simulink model "model"  (Simulink 7.7)
settings: Solver=ode45  StartTime=0.0  StopTime=2500000  FixedStep=0.01  RelTol=1e-3
undefined symbols (not defined in the file): des_figposition
libraries: simeventssink1 x5, simeventsgenerators1 x3, simeventsattributes2 x2, simeventsqueue1 x1, simeventsserver1 x1, simeventsrouting1 x1
settings Model: Creator=Yulia  ModifiedByFormat=Yuli  LastModifiedBy=Yuli  ModifiedComment=Yulia -- Yulia -- Version 1.8
settings Model: ModifiedHistory=|
  | Yulia -- Yulia -- Version 1.8
  | 
  | 
  | Yulia -- Yulia -- Version 1.7
settings OptimizationCC: SimCompilerOptimization=On
settings SimEventsCC: propDiagAttribOutput=1  propDiagFcnCallOutput=1  propDiagStatOutput=0

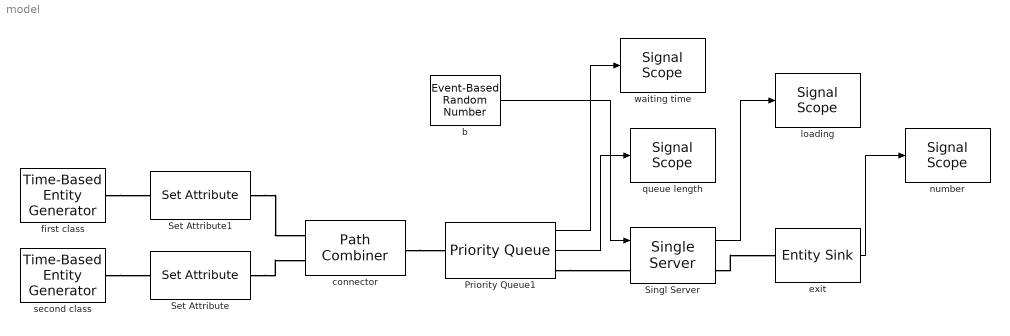
== system model ==
  Priority Queue1 : simeventsqueue1/Priority Queue  Priority=1  SystemSampleTime=-1  Capacity=inf  SortingAttributeName=ServiceTime  SortingDirection=Descending  EnableTOPort=off  StatNumberDeparted=Off  StatNumberInBlock=Off  StatPendingEntity=Off  StatAverageWait=On  StatAverageQueueLength=On  StatNumberTimedout=Off
      settings: AttributesFormatString=Sorting direction =\n%<SortingDirection>
  Set Attribute : simeventsattributes2/Set Attribute  Priority=1  SystemSampleTime=-1  AttributeFrom=Dialog  AttributeName=ServiceTime  AttributeTreatAsVector=1  AttributeValue=2  AttributeCreate=on  StatNumberDeparted=Off  EvaluatedAttributeValue={2}
      settings: AttributesFormatString=ServiceTime = 2\nSwitch = 2
  Set Attribute1 : simeventsattributes2/Set Attribute  Priority=1  SystemSampleTime=-1  AttributeFrom=Dialog  AttributeName=ServiceTime  AttributeTreatAsVector=1  AttributeValue=1  AttributeCreate=on  StatNumberDeparted=Off  EvaluatedAttributeValue={1}
      settings: AttributesFormatString=ServiceTime = 1\nSwitch = 1
  Singl Server : simeventsserver1/Single Server  SystemSampleTime=-1  ServiceTimeFrom=Signal port t  ServiceTime=1  AttributeName=ServiceTime  PriorityServiceCompletion=500  PermitPreemption=off  SortingAttributeName=PriorityAttributeName  SortingDirection=Ascending  WriteToAttribute=off  ResidualAttributeName=ResidualServiceTime  CreateAttribute=on  EnableTOPort=off  StatNumberDeparted=Off  StatNumberInBlock=Off  StatNumberPreempted=Off  StatPendingEntity=Off  StatAverageWait=Off  StatUtilization=On  StatNumberTimedout=Off
  b : simeventsgenerators1/Signal Generators/Event-Based Random Number  SystemSampleTime=-1  distribution=Exponential  meanExp=1  minUnif=1  maxUnif=1  pOneBern=0.25  pSuccessBino=0.5  numTrialBino=1  meanNorm=0  stdNorm=1  minTri=1  maxTri=3  modeTri=2  thresholdLogn=0  scaleLogn=1  shapeLogn=1  pSuccessGeo=0.5  meanPoiss=1  thresholdLogl=0  scaleLogl=1  thresholdGam=0  scaleGam=1  shapeGam=1  minBeta=0  maxBeta=1  shape1Beta=1  shape2Beta=1  minUnid=0  maxUnid=1  numValueUnid=2  thresholdWbl=0  scaleWbl=1  shapeWbl=1  valueVecCont=[0 1]  cdfVecCont=[0 1]  valueVecDisc=[0 1]  probVecDisc=[0.5 0.5]  seed=12345  IsProcessed=on  isConnected=1
  connector : simeventsrouting1/Path Combiner  SystemSampleTime=-1  NumberInputPorts=2  InputPortPrecedence=IN1 port  InitialSeed=45675  SpecifyEventPriority=off  PriorityPathCombinerPortPrecedenceSelection=4100  StatNumberDeparted=Off  StatLastArrivalPort=Off  EvaluatedNumPorts=2
  exit : simeventssink1/Entity Sink  SystemSampleTime=-1  AvailableForArrivals=on  StatNumberArrived=On
  first class : simeventsgenerators1/Entity Generators/Time-Based Entity Generator  SystemSampleTime=-1  GenerateEntitiesUpon=Intergeneration time from dialog  Distribution=Exponential  Minimum=0  Maximum=1  Mean=10  InitialSeed=12345  Period=1  PriorityEntityGeneration=300  GenerateEntityAtSimulationStart=on  ResponseWhenBlocked=Pause generation  ResponseWhenUnblocked=Immediate restart  EntityType=Blank  StatNumberDeparted=Off  StatPendingEntity=Off  StatAverageIntergenerationTime=Off
  loading : simeventssink1/Signal Scope  SystemSampleTime=-1  PlotType=Stair  InputType=Signal  NumInputs=1  AttributeNameY=Count  XInputOptionSignal=Event time  XInputOptionEntity=Event time  AttributeNameX=Count  EnableEntityOutport=on  XMin=0  XMax=10  XLimitExceededOption=Stretch axis limits  YLimitExceededOption=Stretch axis limits  AxisGrid=on  AxisLegend=off  LineDisables=""  LineColors=b  LineStyles=-  LineMarkers=.  OpenScopeAtSimStart=off  Title=""  YLabel=""  XLabel=Time  FigurePosition=des_figposition([5 60 25 25])  AxisZoom=off  DataStoreOption=Limited  DataPointsLimit=10000  StatNumberArrived=Off  ShowCountPlotted=off  ShowToolbar=on
      settings: YMin=0  YMax=10
  number : simeventssink1/Signal Scope  SystemSampleTime=-1  PlotType=Stair  InputType=Signal  NumInputs=1  AttributeNameY=Count  XInputOptionSignal=Event time  XInputOptionEntity=Event time  AttributeNameX=Count  EnableEntityOutport=on  XMin=0  XMax=10  XLimitExceededOption=Stretch axis limits  YLimitExceededOption=Stretch axis limits  AxisGrid=on  AxisLegend=off  LineDisables=""  LineColors=b  LineStyles=-  LineMarkers=.  OpenScopeAtSimStart=off  Title=""  YLabel=""  XLabel=Time  FigurePosition=des_figposition([5 60 25 25])  AxisZoom=off  DataStoreOption=Limited  DataPointsLimit=10000  StatNumberArrived=Off  ShowCountPlotted=off  ShowToolbar=on
      settings: YMin=0  YMax=10
  queue length : simeventssink1/Signal Scope  SystemSampleTime=-1  PlotType=Stair  InputType=Signal  NumInputs=1  AttributeNameY=Count  XInputOptionSignal=Event time  XInputOptionEntity=Event time  AttributeNameX=Count  EnableEntityOutport=on  XMin=0  XMax=10  XLimitExceededOption=Stretch axis limits  YLimitExceededOption=Stretch axis limits  AxisGrid=on  AxisLegend=off  LineDisables=""  LineColors=b  LineStyles=-  LineMarkers=.  OpenScopeAtSimStart=off  Title=""  YLabel=""  XLabel=Time  FigurePosition=des_figposition([5 60 25 25])  AxisZoom=off  DataStoreOption=Limited  DataPointsLimit=10000  StatNumberArrived=Off  ShowCountPlotted=off  ShowToolbar=on
      settings: YMin=0  YMax=10
  second class : simeventsgenerators1/Entity Generators/Time-Based Entity Generator  SystemSampleTime=-1  GenerateEntitiesUpon=Intergeneration time from dialog  Distribution=Exponential  Minimum=0  Maximum=1  Mean=10  InitialSeed=12345  Period=1  PriorityEntityGeneration=300  GenerateEntityAtSimulationStart=on  ResponseWhenBlocked=Pause generation  ResponseWhenUnblocked=Immediate restart  EntityType=Blank  StatNumberDeparted=Off  StatPendingEntity=Off  StatAverageIntergenerationTime=Off
  waiting time : simeventssink1/Signal Scope  SystemSampleTime=-1  PlotType=Stair  InputType=Signal  NumInputs=1  AttributeNameY=Count  XInputOptionSignal=Event time  XInputOptionEntity=Event time  AttributeNameX=Count  EnableEntityOutport=on  XMin=0  XMax=10  XLimitExceededOption=Stretch axis limits  YLimitExceededOption=Stretch axis limits  AxisGrid=on  AxisLegend=off  LineDisables=""  LineColors=b  LineStyles=-  LineMarkers=.  OpenScopeAtSimStart=off  Title=""  YLabel=""  XLabel=Time  FigurePosition=des_figposition([5 60 25 25])  AxisZoom=off  DataStoreOption=Limited  DataPointsLimit=10000  StatNumberArrived=Off  ShowCountPlotted=off  ShowToolbar=on
      settings: YMin=0  YMax=10
  wires:
  b/1 -> Singl Server/1
  Priority Queue1/2 -> queue length/1
  Priority Queue1/1 -> waiting time/1
  exit/1 -> number/1
  Singl Server/1 -> loading/1
  connections:
  Singl Server/RConn1 -- exit/LConn1
  Priority Queue1/RConn1 -- Singl Server/LConn1
  connector/RConn1 -- Priority Queue1/LConn1
  second class/RConn1 -- Set Attribute/LConn1
  first class/RConn1 -- Set Attribute1/LConn1
  Set Attribute/RConn1 -- connector/LConn2
  Set Attribute1/RConn1 -- connector/LConn1
